simulink model "AllMethods"  (R2024a)
settings: Solver=ode4  StartTime=0.0  StopTime=40  FixedStep=dt  RelTol=1e-3
undefined symbols (not defined in the file): a0, a1, a2, a3, a4, a5, a6, a7, A_cplant, Ag, AgN, alpha1, alpha2, B_cplant, C_cplant, C_phys_5dof, CNrt, CRrt, D_cplant, Dd_ss, delay, Ds_ss, dt, dv1, dv2, EQ_intensity, EQ_sw, F, FN, Gnd_ss, Gns_ss, Hs1, Hs2, k3, k4, k6, K_lqr, K_phys_5dof, Kbar_inv, KE, KNbar_inv, Koo, Kot, l, lN, M_phys_5dof, MNrt, Mren, MRrt, Muu, Phi_u2, Rbar, RNbar, Seed_snr
libraries: simulink x4, slpidlib x4, sldrtlib x1
(part 2 of 2)

== system AllMethods/PID控制+坐标变换/坐标转换 此处将横向位移与节点转角转为 两个作动器的位移 ==
  "[x, theta]" : Inport
  Constant : Constant  Value=dv2
  Constant1 : Constant  Value=dv1
  Constant2 : Constant  Value=alpha2
  Constant3 : Constant  Value=alpha1
  Demux1 : Demux  Outputs=2
  Mux : Mux  Inputs=2
  Product : Product
  Product1 : Product
  Sum{,1,3,5} (4 alike) : Sum  Inputs=|++
  Sum2 : Sum  Inputs=|+-
  Sum4 : Sum  Inputs=|+-
  Trigonometric Function{,1..3} (4 alike) : Trigonometry  Operator=cos
  m to mm : Gain  Gain=1000
  "m to mm " : Gain  Gain=1000
  "[xa1,xa2] mm" : Outport  VectorParamsAs1DForOutWhenUnconnected=off
  wires:
  Constant/1 -> Product/1
  Constant2/1 -> Sum1/2, Trigonometric Function1/1
  Sum1/1 -> Trigonometric Function/1
  Trigonometric Function/1 -> Sum2/1
  Trigonometric Function1/1 -> Sum2/2
  Sum2/1 -> Product/2
  Product/1 -> Sum/2
  Sum/1 -> m to mm/1
  Sum4/1 -> Product1/2
  Trigonometric Function3/1 -> Sum4/2
  Trigonometric Function2/1 -> Sum4/1
  Sum3/1 -> Trigonometric Function2/1
  Constant3/1 -> Sum3/2, Trigonometric Function3/1
  Constant1/1 -> Product1/1
  Product1/1 -> Sum5/2
  Sum5/1 -> "m to mm "/1
  "m to mm "/1 -> Mux/1  "xa1 (mm)"
  m to mm/1 -> Mux/2  "xa2 (mm)"
  Demux1/1 -> Sum/1, Sum5/1  "x (m)"
  "[x, theta]"/1 -> Demux1/1
  Demux1/2 -> Sum3/1, Sum1/1  "theta (rad)"
  Mux/1 -> "[xa1,xa2] mm"/1

== system AllMethods/PID控制+坐标变换/控制器与作动器 ==
  Target actuator displacement vector (mm) : Inport
  Control Plant4 : StateSpace  A=A_cplant  B=B_cplant  C=C_cplant  D=D_cplant  InitialCondition=0
  Delay : Delay  DelayLength=37
  Demux7 : Demux  Outputs=2
  Mux4 : Mux  Inputs=2
  PID Controller2 : slpidlib/PID Controller  Controller=PID  Form=Parallel  TimeDomain=Discrete-time  UseExternalTs=off  SampleTime=-1  IntegratorMethod=Forward Euler  FilterMethod=Forward Euler  ControllerParametersSource=internal  P=1  I=50  UseKiTs=off  D=1e-10  UseExternalDerivativeSource=off  N=100  UseFilter=off  TunerSelectOption=Transfer Function Based (PID Tuner App)  InitialConditionSource=internal  InitialConditionForIntegrator=0  InitialConditionForFilter=0  DifferentiatorICPrevScaledInput=0  ExternalReset=none  TrackingMode=off  Kt=1  LimitOutput=off  SatLimitsSource=internal  UpperSaturationLimit=inf  LowerSaturationLimit=-inf  LinearizeAsGain=on  AntiWindupMode=none  Kb=1  LimitIntegrator=off  UpperIntegratorSaturationLimit=inf  LowerIntegratorSaturationLimit=-inf  POutMin=[]  POutMax=[]  IOutMin=[]  IOutMax=[]  DOutMin=[]  DOutMax=[]  NOutMin=[]  NOutMax=[]  SumOutMin=[]  SumOutMax=[]  SaturationOutMin=[]  SaturationOutMax=[]  PParamMin=[]  PParamMax=[]  IParamMin=[]  IParamMax=[]  DParamMin=[]  DParamMax=[]  NParamMin=[]  NParamMax=[]  KbParamMin=[]  KbParamMax=[]  KtParamMin=[]  KtParamMax=[]  KbOutMin=[]  KbOutMax=[]  KtOutMin=[]  KtOutMax=[]  IntegratorOutMin=[]  IntegratorOutMax=[]  FilterOutMin=[]  FilterOutMax=[]  SumI1OutMin=[]  SumI1OutMax=[]  SumI2OutMin=[]  SumI2OutMax=[]  SumI3OutMin=[]  SumI3OutMax=[]  SumI4OutMin=[]  SumI4OutMax=[]  SumDOutMin=[]  SumDOutMax=[]  DifferentiatorOutMin=[]  DifferentiatorOutMax=[]  FilterDiffOutCoefMin=[]  FilterDiffOutCoefMax=[]  ReciprocalOutMin=[]  ReciprocalOutMax=[]  SumDenOutMin=[]  SumDenOutMax=[]  SumNumOutMin=[]  SumNumOutMax=[]  DivideOutMin=[]  DivideOutMax=[]  UdiffTsProdOutMin=[]  UdiffTsProdOutMax=[]  NTsProdOutMin=[]  NTsProdOutMax=[]  UintegralTsProdOutMin=[]  UintegralTsProdOutMax=[]  UngainTsProdOutMin=[]  UngainTsProdOutMax=[]  ClampingZeroOutDataTypeStr=Inherit: Inherit via back propagation  ClampingZeroOutMin=[]  ClampingZeroOutMax=[]  FilterDenConstantOutDataTypeStr=Inherit: Inherit via back propagation  FilterDenConstantOutMin=[]  FilterDenConstantOutMax=[]  PCopyOutDataTypeStr=Inherit: Inherit via back propagation  PCopyOutMin=[]  PCopyOutMax=[]  NCopyOutDataTypeStr=Inherit: Inherit via back propagation  NCopyOutMin=[]  NCopyOutMax=[]  IntegratorContinuousStateAttributes=''  IntegratorStateMustResolveToSignalObject=off  IntegratorRTWStateStorageClass=Auto  FilterContinuousStateAttributes=''  FilterStateMustResolveToSignalObject=off  FilterRTWStateStorageClass=Auto  ParallelPVariant=InternalParameters  IdealPVariant=Disabled  IVariant=InternalParameters  DVariant=InternalParameters  IntegratorVariant=Discrete  SatVariant=Disabled  AWVariant=Passthrough  PCopyVariant=Disabled  TRVariant=Disabled  FdbkBlocksVariant=Forward  IdealPFdbkVariant=Disabled  SatFdbkVariant=Disabled  DerivativeFilterVariant=Differentiator  NVariant=Passthrough  NCopyVariant=Disabled_SignalSpec  FilterICVariant=InternalICsDifferentiator  IntegratorICVariant=InternalICs  ExternalResetVariant=Disabled  TRSumVariant=Passthrough  SumFdbkVariant=Disabled  SumVariant=Sum_PID  TsampFilterVariant=InternalTs  TsampNgainVariant=Passthrough  TsampIntegralVariant=Disabled_SignalSpec  ExternalSaturationOutDataTypeStr=Inherit: Same as second input  DerivativeSourceVariant=ErrorSignal
  PID Controller4 : slpidlib/PID Controller  Controller=PID  Form=Parallel  TimeDomain=Discrete-time  UseExternalTs=off  SampleTime=-1  IntegratorMethod=Forward Euler  FilterMethod=Forward Euler  ControllerParametersSource=internal  P=1  I=50  UseKiTs=off  D=1e-10  UseExternalDerivativeSource=off  N=100  UseFilter=on  TunerSelectOption=Transfer Function Based (PID Tuner App)  InitialConditionSource=internal  InitialConditionForIntegrator=0  InitialConditionForFilter=0  DifferentiatorICPrevScaledInput=0  ExternalReset=none  TrackingMode=off  Kt=1  LimitOutput=off  SatLimitsSource=internal  UpperSaturationLimit=inf  LowerSaturationLimit=-inf  LinearizeAsGain=on  AntiWindupMode=none  Kb=1  LimitIntegrator=off  UpperIntegratorSaturationLimit=inf  LowerIntegratorSaturationLimit=-inf  POutMin=[]  POutMax=[]  IOutMin=[]  IOutMax=[]  DOutMin=[]  DOutMax=[]  NOutMin=[]  NOutMax=[]  SumOutMin=[]  SumOutMax=[]  SaturationOutMin=[]  SaturationOutMax=[]  PParamMin=[]  PParamMax=[]  IParamMin=[]  IParamMax=[]  DParamMin=[]  DParamMax=[]  NParamMin=[]  NParamMax=[]  KbParamMin=[]  KbParamMax=[]  KtParamMin=[]  KtParamMax=[]  KbOutMin=[]  KbOutMax=[]  KtOutMin=[]  KtOutMax=[]  IntegratorOutMin=[]  IntegratorOutMax=[]  FilterOutMin=[]  FilterOutMax=[]  SumI1OutMin=[]  SumI1OutMax=[]  SumI2OutMin=[]  SumI2OutMax=[]  SumI3OutMin=[]  SumI3OutMax=[]  SumI4OutMin=[]  SumI4OutMax=[]  SumDOutMin=[]  SumDOutMax=[]  DifferentiatorOutMin=[]  DifferentiatorOutMax=[]  FilterDiffOutCoefMin=[]  FilterDiffOutCoefMax=[]  ReciprocalOutMin=[]  ReciprocalOutMax=[]  SumDenOutMin=[]  SumDenOutMax=[]  SumNumOutMin=[]  SumNumOutMax=[]  DivideOutMin=[]  DivideOutMax=[]  UdiffTsProdOutMin=[]  UdiffTsProdOutMax=[]  NTsProdOutMin=[]  NTsProdOutMax=[]  UintegralTsProdOutMin=[]  UintegralTsProdOutMax=[]  UngainTsProdOutMin=[]  UngainTsProdOutMax=[]  ClampingZeroOutDataTypeStr=Inherit: Inherit via back propagation  ClampingZeroOutMin=[]  ClampingZeroOutMax=[]  FilterDenConstantOutDataTypeStr=Inherit: Inherit via back propagation  FilterDenConstantOutMin=[]  FilterDenConstantOutMax=[]  PCopyOutDataTypeStr=Inherit: Inherit via back propagation  PCopyOutMin=[]  PCopyOutMax=[]  NCopyOutDataTypeStr=Inherit: Inherit via back propagation  NCopyOutMin=[]  NCopyOutMax=[]  IntegratorContinuousStateAttributes=''  IntegratorStateMustResolveToSignalObject=off  IntegratorRTWStateStorageClass=Auto  FilterContinuousStateAttributes=''  FilterStateMustResolveToSignalObject=off  FilterRTWStateStorageClass=Auto  ParallelPVariant=InternalParameters  IdealPVariant=Disabled  IVariant=InternalParameters  DVariant=InternalParameters  IntegratorVariant=Discrete  SatVariant=Disabled  AWVariant=Passthrough  PCopyVariant=Disabled  TRVariant=Disabled  FdbkBlocksVariant=Forward  IdealPFdbkVariant=Disabled  SatFdbkVariant=Disabled  DerivativeFilterVariant=ForwardEulerFilter  NVariant=InternalParameters  NCopyVariant=Disabled  FilterICVariant=InternalICsFilter  IntegratorICVariant=InternalICs  ExternalResetVariant=Disabled  TRSumVariant=Passthrough  SumFdbkVariant=Disabled  SumVariant=Sum_PID  TsampFilterVariant=InternalTs  TsampNgainVariant=Passthrough  TsampIntegralVariant=Disabled_SignalSpec  ExternalSaturationOutDataTypeStr=Inherit: Same as second input  DerivativeSourceVariant=ErrorSignal
  Sum11 : Sum  Inputs=|+-
  Filtered actuator displacement vector : Outport
  wires:
  PID Controller4/1 -> Mux4/2
  Control Plant4/1 -> Delay/1, Filtered actuator displacement vector/1  "Filtered actuator displacement vector"
  Sum11/1 -> Demux7/1
  PID Controller2/1 -> Mux4/1
  Mux4/1 -> Control Plant4/1
  Target actuator displacement vector (mm)/1 -> Sum11/1
  Demux7/1 -> PID Controller2/1
  Demux7/2 -> PID Controller4/1
  Delay/1 -> Sum11/2

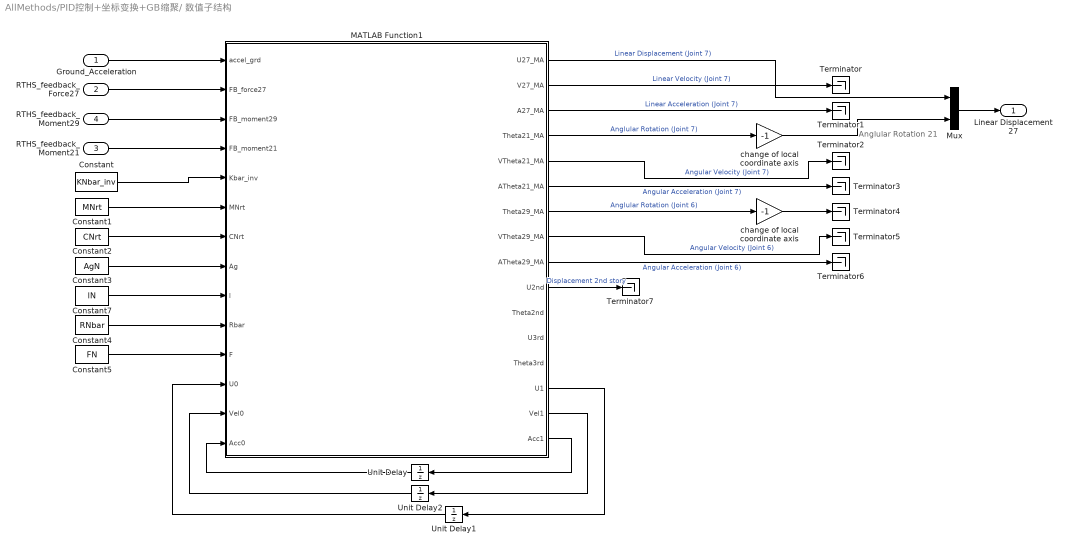
== system AllMethods/PID控制+坐标变换+GB缩聚/ 数值子结构 ==
  note: Anglular Rotation 21
  Ground_Acceleration : Inport
  RTHS_feedback_Force27 : Inport  Port=2
  RTHS_feedback_Moment21 : Inport  Port=3
  RTHS_feedback_Moment29 : Inport  Port=4
  Constant : Constant  Value=KNbar_inv  VectorParams1D=off
  Constant1 : Constant  Value=MNrt  VectorParams1D=off
  Constant2 : Constant  Value=CNrt  VectorParams1D=off
  Constant3 : Constant  Value=AgN  VectorParams1D=off
  Constant4 : Constant  Value=RNbar  VectorParams1D=off
  Constant5 : Constant  Value=FN  VectorParams1D=off
  Constant7 : Constant  Value=lN  VectorParams1D=off
  MATLAB Function1 : MATLAB Function  TreatAsAtomicUnit=on
  Mux : Mux  Inputs=2
  Terminator{,1..7} (8 alike) : Terminator
  Unit Delay : UnitDelay  SampleTime=-1  HasFrameUpgradeWarning=on
  Unit Delay1 : UnitDelay  SampleTime=-1  HasFrameUpgradeWarning=on
  Unit Delay2 : UnitDelay  SampleTime=-1  HasFrameUpgradeWarning=on
  change of local coordinate axis : Gain  Gain=-1
  "change of local coordinate axis  " : Gain  Gain=-1
  Linear Displacement 27 : Outport  VectorParamsAs1DForOutWhenUnconnected=off
  wires:
  Ground_Acceleration/1 -> MATLAB Function1/1(accel_grd)
  RTHS_feedback_Force27/1 -> MATLAB Function1/2(FB_force27)
  RTHS_feedback_Moment29/1 -> MATLAB Function1/3(FB_moment29)
  MATLAB Function1/1(U27_MA) -> Mux/1  "Linear Displacement (Joint 7)"
  MATLAB Function1/4(Theta21_MA) -> change of local coordinate axis/1  "Anglular Rotation (Joint 7)"
  Constant/1 -> MATLAB Function1/5(Kbar_inv)
  Constant1/1 -> MATLAB Function1/6(MNrt)
  Constant2/1 -> MATLAB Function1/7(CNrt)
  Constant3/1 -> MATLAB Function1/8(Ag)
  Constant7/1 -> MATLAB Function1/9(l)
  Constant4/1 -> MATLAB Function1/10(Rbar)
  Unit Delay1/1 -> MATLAB Function1/12(U0)
  Unit Delay2/1 -> MATLAB Function1/13(Vel0)
  Unit Delay/1 -> MATLAB Function1/14(Acc0)
  MATLAB Function1/15(Vel1) -> Unit Delay2/1
  MATLAB Function1/16(Acc1) -> Unit Delay/1
  MATLAB Function1/14(U1) -> Unit Delay1/1
  Constant5/1 -> MATLAB Function1/11(F)
  MATLAB Function1/2(V27_MA) -> Terminator/1  "Linear Velocity (Joint 7)"
  MATLAB Function1/3(A27_MA) -> Terminator1/1  "Linear Acceleration (Joint 7)"
  MATLAB Function1/5(VTheta21_MA) -> Terminator2/1  "Angular Velocity (Joint 7)"
  MATLAB Function1/6(ATheta21_MA) -> Terminator3/1  "Angular Acceleration (Joint 7)"
  MATLAB Function1/9(ATheta29_MA) -> Terminator6/1  "Angular Acceleration (Joint 6)"
  MATLAB Function1/8(VTheta29_MA) -> Terminator5/1  "Angular Velocity (Joint 6)"
  MATLAB Function1/7(Theta29_MA) -> "change of local coordinate axis  "/1  "Anglular Rotation (Joint 6)"
  RTHS_feedback_Moment21/1 -> MATLAB Function1/4(FB_moment21)
  change of local coordinate axis/1 -> Mux/2
  "change of local coordinate axis  "/1 -> Terminator4/1
  Mux/1 -> Linear Displacement 27/1
  MATLAB Function1/10(U2nd) -> Terminator7/1  "Displacement 2nd story"

== system AllMethods/PID控制+坐标变换+GB缩聚/Feedback Force Computation ==
  note: F(27)
  note: M(21)
  note: M(29)
  "[x_est, theta_est] (m,rad)" : Inport
  Demux : Demux  Outputs=3
  Derivative : Derivative
  Derivative1 : Derivative
  Gain1 : Gain  Gain=K_phys_5dof  Multiplication=Matrix(K*u) (u vector)
  Gain2 : Gain  Gain=C_phys_5dof  Multiplication=Matrix(K*u) (u vector)
  Gain3 : Gain  Gain=M_phys_5dof  Multiplication=Matrix(K*u) (u vector)
  Gain4 : Gain  Commented=on  Gain=-inv(Koo)*Kot  Multiplication=Matrix(K*u) (u vector)
  Mux2 : Mux  Commented=on  Inputs=2
  Mux3 : Mux  Inputs=2
  Selector : Selector  InputPortWidth=5  IndexOptions=Index vector (dialog)  Indices=[1 2 3]  OutputSizes=1
  Sum : Sum  Inputs=+|+|+
  Sum1 : Sum  Inputs=|++
  change of local coordinate axis2 : Gain  Gain=-1
  change of local coordinate axis3 : Gain  Gain=-1
  动态位移 : Gain  Gain=Phi_u2*Phi_u2' * Muu  Multiplication=Matrix(K*u) (u vector)
  静态位移 : Gain  Gain=-Kuu \ Kuc  Multiplication=Matrix(K*u) (u vector)
  F(27)_phys (N) : Outport  VectorParamsAs1DForOutWhenUnconnected=off
  M(21)_phys (N*m) : Outport  Port=2  VectorParamsAs1DForOutWhenUnconnected=off
  M(29)_phys (N*m) : Outport  Port=3  VectorParamsAs1DForOutWhenUnconnected=off
  wires:
  Derivative1/1 -> Gain3/1
  Gain2/1 -> Sum/2
  Derivative/1 -> Gain2/1, Derivative1/1
  Gain1/1 -> Sum/1
  Demux/1 -> F(27)_phys (N)/1
  Sum/1 -> Selector/1
  Selector/1 -> Demux/1
  Gain3/1 -> Sum/3
  Demux/2 -> change of local coordinate axis2/1
  Demux/3 -> change of local coordinate axis3/1
  Mux3/1 -> Derivative/1, Gain1/1
  change of local coordinate axis2/1 -> M(21)_phys (N*m)/1
  change of local coordinate axis3/1 -> M(29)_phys (N*m)/1
  静态位移/1 -> 动态位移/1, Sum1/2
  "[x_est, theta_est] (m,rad)"/1 -> Mux2/1, Gain4/1, Mux3/1, 静态位移/1
  动态位移/1 -> Sum1/1
  Gain4/1 -> Mux2/2
  Sum1/1 -> Mux3/2

== system AllMethods/PID控制+坐标变换+GB缩聚/坐标转换 此处将两个作动器的位移转为 横向位移与节点转角  ==
  "[xm1_est, xm2_est] (mm)" : Inport
  Constant : Constant  Value=dv2
  Constant1 : Constant  Value=dv1
  Constant2 : Constant  Value=alpha2
  Constant3 : Constant  Value=alpha1
  Demux1 : Demux  Outputs=2
  Divide : Product  Inputs=*/
  Gain : Gain  Gain=2
  Mux2 : Mux  Inputs=2
  Product : Product
  Product1 : Product
  Sum : Sum  Inputs=+-|
  Sum1 : Sum  Inputs=|++
  Sum2 : Sum  Inputs=|+-
  Sum3 : Sum  Inputs=-+|
  Trigonometric Function1 : Trigonometry
  Trigonometric Function2 : Trigonometry  Operator=cos
  Trigonometric Function3 : Trigonometry  Operator=cos
  Trigonometric Function4 : Trigonometry  Operator=asin
  mm to m : Gain  Gain=1/1000
  "mm to m " : Gain  Gain=1/1000
  "[x, theta] (m, rad)" : Outport  VectorParamsAs1DForOutWhenUnconnected=off
  wires:
  Constant2/1 -> Trigonometric Function1/1
  Constant1/1 -> Product1/1
  Demux1/1 -> mm to m/1
  Demux1/2 -> "mm to m "/1
  Sum/1 -> Divide/1
  Constant/1 -> Gain/1
  Trigonometric Function1/1 -> Product/2
  Gain/1 -> Product/1
  Product/1 -> Divide/2
  Divide/1 -> Sum1/2, Trigonometric Function4/1
  Sum1/1 -> Trigonometric Function2/1
  Constant3/1 -> Sum1/1, Trigonometric Function3/1
  Sum3/1 -> Product1/2
  Sum2/1 -> Mux2/1
  Trigonometric Function2/1 -> Sum3/2
  Trigonometric Function3/1 -> Sum3/1
  Product1/1 -> Sum2/2
  mm to m/1 -> Sum2/1, Sum/1
  "mm to m "/1 -> Sum/2
  Trigonometric Function4/1 -> Mux2/2
  "[xm1_est, xm2_est] (mm)"/1 -> Demux1/1
  Mux2/1 -> "[x, theta] (m, rad)"/1

== system AllMethods/PID控制+坐标变换+GB缩聚/坐标转换 此处将横向位移与节点转角转为 两个作动器的位移 ==
  "[x, theta]" : Inport
  Constant : Constant  Value=dv2
  Constant1 : Constant  Value=dv1
  Constant2 : Constant  Value=alpha2
  Constant3 : Constant  Value=alpha1
  Demux1 : Demux  Outputs=2
  Mux : Mux  Inputs=2
  Product : Product
  Product1 : Product
  Sum{,1,3,5} (4 alike) : Sum  Inputs=|++
  Sum2 : Sum  Inputs=|+-
  Sum4 : Sum  Inputs=|+-
  Trigonometric Function{,1..3} (4 alike) : Trigonometry  Operator=cos
  m to mm : Gain  Gain=1000
  "m to mm " : Gain  Gain=1000
  "[xa1,xa2] mm" : Outport  VectorParamsAs1DForOutWhenUnconnected=off
  wires:
  Constant/1 -> Product/1
  Constant2/1 -> Sum1/2, Trigonometric Function1/1
  Sum1/1 -> Trigonometric Function/1
  Trigonometric Function/1 -> Sum2/1
  Trigonometric Function1/1 -> Sum2/2
  Sum2/1 -> Product/2
  Product/1 -> Sum/2
  Sum/1 -> m to mm/1
  Sum4/1 -> Product1/2
  Trigonometric Function3/1 -> Sum4/2
  Trigonometric Function2/1 -> Sum4/1
  Sum3/1 -> Trigonometric Function2/1
  Constant3/1 -> Sum3/2, Trigonometric Function3/1
  Constant1/1 -> Product1/1
  Product1/1 -> Sum5/2
  Sum5/1 -> "m to mm "/1
  "m to mm "/1 -> Mux/1  "xa1 (mm)"
  m to mm/1 -> Mux/2  "xa2 (mm)"
  Demux1/1 -> Sum/1, Sum5/1  "x (m)"
  "[x, theta]"/1 -> Demux1/1
  Demux1/2 -> Sum3/1, Sum1/1  "theta (rad)"
  Mux/1 -> "[xa1,xa2] mm"/1

== system AllMethods/PID控制+坐标变换+GB缩聚/控制器与作动器 ==
  Target actuator displacement vector (mm) : Inport
  Control Plant4 : StateSpace  A=A_cplant  B=B_cplant  C=C_cplant  D=D_cplant  InitialCondition=0
  Delay : Delay  DelayLength=37
  Demux7 : Demux  Outputs=2
  Mux4 : Mux  Inputs=2
  PID Controller2 : slpidlib/PID Controller  Controller=PID  Form=Parallel  TimeDomain=Discrete-time  UseExternalTs=off  SampleTime=-1  IntegratorMethod=Forward Euler  FilterMethod=Forward Euler  ControllerParametersSource=internal  P=1  I=50  UseKiTs=off  D=1e-10  UseExternalDerivativeSource=off  N=100  UseFilter=off  TunerSelectOption=Transfer Function Based (PID Tuner App)  InitialConditionSource=internal  InitialConditionForIntegrator=0  InitialConditionForFilter=0  DifferentiatorICPrevScaledInput=0  ExternalReset=none  TrackingMode=off  Kt=1  LimitOutput=off  SatLimitsSource=internal  UpperSaturationLimit=inf  LowerSaturationLimit=-inf  LinearizeAsGain=on  AntiWindupMode=none  Kb=1  LimitIntegrator=off  UpperIntegratorSaturationLimit=inf  LowerIntegratorSaturationLimit=-inf  POutMin=[]  POutMax=[]  IOutMin=[]  IOutMax=[]  DOutMin=[]  DOutMax=[]  NOutMin=[]  NOutMax=[]  SumOutMin=[]  SumOutMax=[]  SaturationOutMin=[]  SaturationOutMax=[]  PParamMin=[]  PParamMax=[]  IParamMin=[]  IParamMax=[]  DParamMin=[]  DParamMax=[]  NParamMin=[]  NParamMax=[]  KbParamMin=[]  KbParamMax=[]  KtParamMin=[]  KtParamMax=[]  KbOutMin=[]  KbOutMax=[]  KtOutMin=[]  KtOutMax=[]  IntegratorOutMin=[]  IntegratorOutMax=[]  FilterOutMin=[]  FilterOutMax=[]  SumI1OutMin=[]  SumI1OutMax=[]  SumI2OutMin=[]  SumI2OutMax=[]  SumI3OutMin=[]  SumI3OutMax=[]  SumI4OutMin=[]  SumI4OutMax=[]  SumDOutMin=[]  SumDOutMax=[]  DifferentiatorOutMin=[]  DifferentiatorOutMax=[]  FilterDiffOutCoefMin=[]  FilterDiffOutCoefMax=[]  ReciprocalOutMin=[]  ReciprocalOutMax=[]  SumDenOutMin=[]  SumDenOutMax=[]  SumNumOutMin=[]  SumNumOutMax=[]  DivideOutMin=[]  DivideOutMax=[]  UdiffTsProdOutMin=[]  UdiffTsProdOutMax=[]  NTsProdOutMin=[]  NTsProdOutMax=[]  UintegralTsProdOutMin=[]  UintegralTsProdOutMax=[]  UngainTsProdOutMin=[]  UngainTsProdOutMax=[]  ClampingZeroOutDataTypeStr=Inherit: Inherit via back propagation  ClampingZeroOutMin=[]  ClampingZeroOutMax=[]  FilterDenConstantOutDataTypeStr=Inherit: Inherit via back propagation  FilterDenConstantOutMin=[]  FilterDenConstantOutMax=[]  PCopyOutDataTypeStr=Inherit: Inherit via back propagation  PCopyOutMin=[]  PCopyOutMax=[]  NCopyOutDataTypeStr=Inherit: Inherit via back propagation  NCopyOutMin=[]  NCopyOutMax=[]  IntegratorContinuousStateAttributes=''  IntegratorStateMustResolveToSignalObject=off  IntegratorRTWStateStorageClass=Auto  FilterContinuousStateAttributes=''  FilterStateMustResolveToSignalObject=off  FilterRTWStateStorageClass=Auto  ParallelPVariant=InternalParameters  IdealPVariant=Disabled  IVariant=InternalParameters  DVariant=InternalParameters  IntegratorVariant=Discrete  SatVariant=Disabled  AWVariant=Passthrough  PCopyVariant=Disabled  TRVariant=Disabled  FdbkBlocksVariant=Forward  IdealPFdbkVariant=Disabled  SatFdbkVariant=Disabled  DerivativeFilterVariant=Differentiator  NVariant=Passthrough  NCopyVariant=Disabled_SignalSpec  FilterICVariant=InternalICsDifferentiator  IntegratorICVariant=InternalICs  ExternalResetVariant=Disabled  TRSumVariant=Passthrough  SumFdbkVariant=Disabled  SumVariant=Sum_PID  TsampFilterVariant=InternalTs  TsampNgainVariant=Passthrough  TsampIntegralVariant=Disabled_SignalSpec  ExternalSaturationOutDataTypeStr=Inherit: Same as second input  DerivativeSourceVariant=ErrorSignal
  PID Controller4 : slpidlib/PID Controller  Controller=PID  Form=Parallel  TimeDomain=Discrete-time  UseExternalTs=off  SampleTime=-1  IntegratorMethod=Forward Euler  FilterMethod=Forward Euler  ControllerParametersSource=internal  P=1  I=50  UseKiTs=off  D=1e-10  UseExternalDerivativeSource=off  N=100  UseFilter=on  TunerSelectOption=Transfer Function Based (PID Tuner App)  InitialConditionSource=internal  InitialConditionForIntegrator=0  InitialConditionForFilter=0  DifferentiatorICPrevScaledInput=0  ExternalReset=none  TrackingMode=off  Kt=1  LimitOutput=off  SatLimitsSource=internal  UpperSaturationLimit=inf  LowerSaturationLimit=-inf  LinearizeAsGain=on  AntiWindupMode=none  Kb=1  LimitIntegrator=off  UpperIntegratorSaturationLimit=inf  LowerIntegratorSaturationLimit=-inf  POutMin=[]  POutMax=[]  IOutMin=[]  IOutMax=[]  DOutMin=[]  DOutMax=[]  NOutMin=[]  NOutMax=[]  SumOutMin=[]  SumOutMax=[]  SaturationOutMin=[]  SaturationOutMax=[]  PParamMin=[]  PParamMax=[]  IParamMin=[]  IParamMax=[]  DParamMin=[]  DParamMax=[]  NParamMin=[]  NParamMax=[]  KbParamMin=[]  KbParamMax=[]  KtParamMin=[]  KtParamMax=[]  KbOutMin=[]  KbOutMax=[]  KtOutMin=[]  KtOutMax=[]  IntegratorOutMin=[]  IntegratorOutMax=[]  FilterOutMin=[]  FilterOutMax=[]  SumI1OutMin=[]  SumI1OutMax=[]  SumI2OutMin=[]  SumI2OutMax=[]  SumI3OutMin=[]  SumI3OutMax=[]  SumI4OutMin=[]  SumI4OutMax=[]  SumDOutMin=[]  SumDOutMax=[]  DifferentiatorOutMin=[]  DifferentiatorOutMax=[]  FilterDiffOutCoefMin=[]  FilterDiffOutCoefMax=[]  ReciprocalOutMin=[]  ReciprocalOutMax=[]  SumDenOutMin=[]  SumDenOutMax=[]  SumNumOutMin=[]  SumNumOutMax=[]  DivideOutMin=[]  DivideOutMax=[]  UdiffTsProdOutMin=[]  UdiffTsProdOutMax=[]  NTsProdOutMin=[]  NTsProdOutMax=[]  UintegralTsProdOutMin=[]  UintegralTsProdOutMax=[]  UngainTsProdOutMin=[]  UngainTsProdOutMax=[]  ClampingZeroOutDataTypeStr=Inherit: Inherit via back propagation  ClampingZeroOutMin=[]  ClampingZeroOutMax=[]  FilterDenConstantOutDataTypeStr=Inherit: Inherit via back propagation  FilterDenConstantOutMin=[]  FilterDenConstantOutMax=[]  PCopyOutDataTypeStr=Inherit: Inherit via back propagation  PCopyOutMin=[]  PCopyOutMax=[]  NCopyOutDataTypeStr=Inherit: Inherit via back propagation  NCopyOutMin=[]  NCopyOutMax=[]  IntegratorContinuousStateAttributes=''  IntegratorStateMustResolveToSignalObject=off  IntegratorRTWStateStorageClass=Auto  FilterContinuousStateAttributes=''  FilterStateMustResolveToSignalObject=off  FilterRTWStateStorageClass=Auto  ParallelPVariant=InternalParameters  IdealPVariant=Disabled  IVariant=InternalParameters  DVariant=InternalParameters  IntegratorVariant=Discrete  SatVariant=Disabled  AWVariant=Passthrough  PCopyVariant=Disabled  TRVariant=Disabled  FdbkBlocksVariant=Forward  IdealPFdbkVariant=Disabled  SatFdbkVariant=Disabled  DerivativeFilterVariant=ForwardEulerFilter  NVariant=InternalParameters  NCopyVariant=Disabled  FilterICVariant=InternalICsFilter  IntegratorICVariant=InternalICs  ExternalResetVariant=Disabled  TRSumVariant=Passthrough  SumFdbkVariant=Disabled  SumVariant=Sum_PID  TsampFilterVariant=InternalTs  TsampNgainVariant=Passthrough  TsampIntegralVariant=Disabled_SignalSpec  ExternalSaturationOutDataTypeStr=Inherit: Same as second input  DerivativeSourceVariant=ErrorSignal
  Sum11 : Sum  Inputs=|+-
  Filtered actuator displacement vector : Outport
  wires:
  PID Controller4/1 -> Mux4/2
  Control Plant4/1 -> Delay/1, Filtered actuator displacement vector/1  "Filtered actuator displacement vector"
  Sum11/1 -> Demux7/1
  PID Controller2/1 -> Mux4/1
  Mux4/1 -> Control Plant4/1
  Target actuator displacement vector (mm)/1 -> Sum11/1
  Demux7/1 -> PID Controller2/1
  Demux7/2 -> PID Controller4/1
  Delay/1 -> Sum11/2

== system AllMethods/离散时间下封装模块/Feedback Force Computation ==
  "[x_est, theta_est] (m,rad)" : Inport
  Derivative : Derivative
  Derivative1 : Derivative
  Gain1 : Gain  Gain=K_phys_5dof  Multiplication=Matrix(K*u) (u vector)
  Gain2 : Gain  Gain=C_phys_5dof  Multiplication=Matrix(K*u) (u vector)
  Gain3 : Gain  Gain=M_phys_5dof  Multiplication=Matrix(K*u) (u vector)
  Sum : Sum  Inputs=+|+|+
  F(27)_phys (N) : Outport  VectorParamsAs1DForOutWhenUnconnected=off
  wires:
  Derivative1/1 -> Gain3/1
  Gain2/1 -> Sum/2
  Derivative/1 -> Gain2/1, Derivative1/1
  Gain1/1 -> Sum/1
  Sum/1 -> F(27)_phys (N)/1
  Gain3/1 -> Sum/3
  "[x_est, theta_est] (m,rad)"/1 -> Derivative/1, Gain1/1

== system AllMethods/连续时间下封装模块/Feedback Force Computation1 ==
  "[x_est, theta_est] (m,rad)" : Inport
  Derivative : Derivative
  Derivative1 : Derivative
  Gain1 : Gain  Gain=K_phys_5dof  Multiplication=Matrix(K*u) (u vector)
  Gain2 : Gain  Gain=C_phys_5dof  Multiplication=Matrix(K*u) (u vector)
  Gain3 : Gain  Gain=M_phys_5dof  Multiplication=Matrix(K*u) (u vector)
  Sum : Sum  Inputs=+|+|+
  F(27)_phys (N) : Outport  VectorParamsAs1DForOutWhenUnconnected=off
  wires:
  Derivative1/1 -> Gain3/1
  Gain2/1 -> Sum/2
  Derivative/1 -> Gain2/1, Derivative1/1
  Gain1/1 -> Sum/1
  Sum/1 -> F(27)_phys (N)/1
  Gain3/1 -> Sum/3
  "[x_est, theta_est] (m,rad)"/1 -> Derivative/1, Gain1/1

== matlab function AllMethods/LQG+坐标变换+GB缩聚/ NUMERICAL SUBSTRUCTURE/MATLAB Function1 ==
  data: U27_MA output; V27_MA output; A27_MA output; Theta21_MA output; VTheta21_MA output; ATheta21_MA output; Theta29_MA output; VTheta29_MA output; ATheta29_MA output; U2nd output; Theta2nd output; U3rd output; Theta3rd output; U1 output; Vel1 output; Acc1 output; accel_grd input; FB_force27 input; FB_moment29 input; FB_moment21 input; Kbar_inv input; MNrt input; CNrt input; Ag input; l input; Rbar input; F input; U0 input; Vel0 input; Acc0 input; a0 parameter; a1 parameter; a2 parameter; a3 parameter; a4 parameter; a5 parameter; a6 parameter; a7 parameter
function [U27_MA,V27_MA,A27_MA,Theta21_MA,VTheta21_MA,ATheta21_MA,Theta29_MA,VTheta29_MA,ATheta29_MA,U2nd,Theta2nd,U3rd,Theta3rd,U1,Vel1,Acc1]=...
    fcn(accel_grd,FB_force27,FB_moment29,FB_moment21,Kbar_inv, MNrt, CNrt,Ag,l,Rbar,F,...
    U0,Vel0,Acc0, a0, a1, a2, a3, a4, a5, a6, a7)
             
             
    % ============================
	% *  Update next iteration   *
	% ============================
    ndof = length(Kbar_inv);
    U1   = zeros(ndof,1);
    Vel1 = zeros(ndof,1);
    Acc1 = zeros(ndof,1);
    
    U27_MA = 0;
    V27_MA = 0;
    A27_MA = 0;

    Theta21_MA = 0;
    VTheta21_MA = 0;
    ATheta21_MA = 0;
% 
%     U6_MA = 0;
%     V6_MA = 0;
%     A6_MA = 0;
    U2nd = 0 ;              %Displacement 2nd story, node 12, DOF 26
    Theta2nd = 0;          %Rotation 2nd story, node 12, DOF 22
    U3rd = 0;              %Displacement 3rd story, node 16, DOF 13
    Theta3rd = 0;           %Rotation 3rd story, node 16, DOF 3


    Theta29_MA = 0;
    VTheta29_MA = 0;
    ATheta29_MA = 0;

    % ============================
	% *  Feedback Force / Moment *
	% ============================
    F(27) = FB_force27;
    F(21) = FB_moment21;
    F(29) = FB_moment29;

    % ==========================
	% *     Update Matrices    *
	% ==========================
    Ag(:)  = accel_grd * l;
    
   	% ==========================
	% * 	  Form Rbar  	   *
	% ==========================
	Rbar = ( (MNrt * ((a0*U0)+(a2*Vel0)+(a3*Acc0))) + ...
		     (CNrt * ((a1*U0)+(a4*Vel0)+(a5*Acc0))) - F - (MNrt * Ag) );
    
    % ==========================
	% * Solve for Displacement *
	% ==========================
	U1 = Kbar_inv * Rbar;
    
	% ============================
	% * Compute Velocity & Accel *
	% ============================
	Acc1=a0*(U1-U0)-a2*Vel0-a3*Acc0;
	Vel1=Vel0+a7*Acc1+a6*Acc0; 

	% ============================
	% *    Output u1 and theta   *
	% ============================
    U27_MA    = U1(27);
    V27_MA    = Vel1(27);
    A27_MA    = Acc1(27);    

%     U6_MA    = U1(27);
%     V6_MA    = Vel1(27);
%     A6_MA    = Acc1(27);

    Theta21_MA = U1(21);
    VTheta21_MA = Vel1(21);
    ATheta21_MA = Acc1(21);

    Theta29_MA = U1(29);
    VTheta29_MA = Vel1(29);
    ATheta29_MA = Acc1(29);
    
    % ADDED by Johnny
    U2nd = U1(26);              %Displacement 2nd story, node 12, DOF 26
    Theta2nd = U1(22);          %Rotation 2nd story, node 12, DOF 22
    U3rd = U1(13);              %Displacement 3rd story, node 16, DOF 13
    Theta3rd = U1(3);           %Rotation 3rd story, node 16, DOF 3

end

== matlab function AllMethods/LQG+坐标变换/ NUMERICAL SUBSTRUCTURE/MATLAB Function1 ==
  data: U27_MA output; V27_MA output; A27_MA output; Theta21_MA output; VTheta21_MA output; ATheta21_MA output; Theta29_MA output; VTheta29_MA output; ATheta29_MA output; U2nd output; Theta2nd output; U3rd output; Theta3rd output; U1 output; Vel1 output; Acc1 output; accel_grd input; FB_force27 input; FB_moment29 input; FB_moment21 input; Kbar_inv input; MNrt input; CNrt input; Ag input; l input; Rbar input; F input; U0 input; Vel0 input; Acc0 input; a0 parameter; a1 parameter; a2 parameter; a3 parameter; a4 parameter; a5 parameter; a6 parameter; a7 parameter
function [U27_MA,V27_MA,A27_MA,Theta21_MA,VTheta21_MA,ATheta21_MA,Theta29_MA,VTheta29_MA,ATheta29_MA,U2nd,Theta2nd,U3rd,Theta3rd,U1,Vel1,Acc1]=...
    fcn(accel_grd,FB_force27,FB_moment29,FB_moment21,Kbar_inv, MNrt, CNrt,Ag,l,Rbar,F,...
    U0,Vel0,Acc0, a0, a1, a2, a3, a4, a5, a6, a7)
             
             
    % ============================
	% *  Update next iteration   *
	% ============================
    ndof = length(Kbar_inv);
    U1   = zeros(ndof,1);
    Vel1 = zeros(ndof,1);
    Acc1 = zeros(ndof,1);
    
    U27_MA = 0;
    V27_MA = 0;
    A27_MA = 0;

    Theta21_MA = 0;
    VTheta21_MA = 0;
    ATheta21_MA = 0;
% 
%     U6_MA = 0;
%     V6_MA = 0;
%     A6_MA = 0;
    U2nd = 0 ;              %Displacement 2nd story, node 12, DOF 26
    Theta2nd = 0;          %Rotation 2nd story, node 12, DOF 22
    U3rd = 0;              %Displacement 3rd story, node 16, DOF 13
    Theta3rd = 0;           %Rotation 3rd story, node 16, DOF 3


    Theta29_MA = 0;
    VTheta29_MA = 0;
    ATheta29_MA = 0;

    % ============================
	% *  Feedback Force / Moment *
	% ============================
    F(27) = FB_force27;
    F(21) = FB_moment21;
    F(29) = FB_moment29;

    % ==========================
	% *     Update Matrices    *
	% ==========================
    Ag(:)  = accel_grd * l;
    
   	% ==========================
	% * 	  Form Rbar  	   *
	% ==========================
	Rbar = ( (MNrt * ((a0*U0)+(a2*Vel0)+(a3*Acc0))) + ...
		     (CNrt * ((a1*U0)+(a4*Vel0)+(a5*Acc0))) - F - (MNrt * Ag) );
    
    % ==========================
	% * Solve for Displacement *
	% ==========================
	U1 = Kbar_inv * Rbar;
    
	% ============================
	% * Compute Velocity & Accel *
	% ============================
	Acc1=a0*(U1-U0)-a2*Vel0-a3*Acc0;
	Vel1=Vel0+a7*Acc1+a6*Acc0; 

	% ============================
	% *    Output u1 and theta   *
	% ============================
    U27_MA    = U1(27);
    V27_MA    = Vel1(27);
    A27_MA    = Acc1(27);    

%     U6_MA    = U1(27);
%     V6_MA    = Vel1(27);
%     A6_MA    = Acc1(27);

    Theta21_MA = U1(21);
    VTheta21_MA = Vel1(21);
    ATheta21_MA = Acc1(21);

    Theta29_MA = U1(29);
    VTheta29_MA = Vel1(29);
    ATheta29_MA = Acc1(29);
    
    % ADDED by Johnny
    U2nd = U1(26);              %Displacement 2nd story, node 12, DOF 26
    Theta2nd = U1(22);          %Rotation 2nd story, node 12, DOF 22
    U3rd = U1(13);              %Displacement 3rd story, node 16, DOF 13
    Theta3rd = U1(3);           %Rotation 3rd story, node 16, DOF 3

end

== matlab function AllMethods/PID控制+坐标变换+GB缩聚/ 数值子结构/MATLAB Function1 ==
  data: U27_MA output; V27_MA output; A27_MA output; Theta21_MA output; VTheta21_MA output; ATheta21_MA output; Theta29_MA output; VTheta29_MA output; ATheta29_MA output; U2nd output; Theta2nd output; U3rd output; Theta3rd output; U1 output; Vel1 output; Acc1 output; accel_grd input; FB_force27 input; FB_moment29 input; FB_moment21 input; Kbar_inv input; MNrt input; CNrt input; Ag input; l input; Rbar input; F input; U0 input; Vel0 input; Acc0 input; a0 parameter; a1 parameter; a2 parameter; a3 parameter; a4 parameter; a5 parameter; a6 parameter; a7 parameter
function [U27_MA,V27_MA,A27_MA,Theta21_MA,VTheta21_MA,ATheta21_MA,Theta29_MA,VTheta29_MA,ATheta29_MA,U2nd,Theta2nd,U3rd,Theta3rd,U1,Vel1,Acc1]=...
    fcn(accel_grd,FB_force27,FB_moment29,FB_moment21,Kbar_inv, MNrt, CNrt,Ag,l,Rbar,F,...
    U0,Vel0,Acc0, a0, a1, a2, a3, a4, a5, a6, a7)
             
             
    % ============================
	% *  Update next iteration   *
	% ============================
    ndof = length(Kbar_inv);
    U1   = zeros(ndof,1);
    Vel1 = zeros(ndof,1);
    Acc1 = zeros(ndof,1);
    
    U27_MA = 0;
    V27_MA = 0;
    A27_MA = 0;

    Theta21_MA = 0;
    VTheta21_MA = 0;
    ATheta21_MA = 0;
% 
%     U6_MA = 0;
%     V6_MA = 0;
%     A6_MA = 0;
    U2nd = 0 ;              %Displacement 2nd story, node 12, DOF 26
    Theta2nd = 0;          %Rotation 2nd story, node 12, DOF 22
    U3rd = 0;              %Displacement 3rd story, node 16, DOF 13
    Theta3rd = 0;           %Rotation 3rd story, node 16, DOF 3


    Theta29_MA = 0;
    VTheta29_MA = 0;
    ATheta29_MA = 0;

    % ============================
	% *  Feedback Force / Moment *
	% ============================
    F(27) = FB_force27;
    F(21) = FB_moment21;
    F(29) = FB_moment29;

    % ==========================
	% *     Update Matrices    *
	% ==========================
    Ag(:)  = accel_grd * l;
    
   	% ==========================
	% * 	  Form Rbar  	   *
	% ==========================
	Rbar = ( (MNrt * ((a0*U0)+(a2*Vel0)+(a3*Acc0))) + ...
		     (CNrt * ((a1*U0)+(a4*Vel0)+(a5*Acc0))) - F - (MNrt * Ag) );
    
    % ==========================
	% * Solve for Displacement *
	% ==========================
	U1 = Kbar_inv * Rbar;
    
	% ============================
	% * Compute Velocity & Accel *
	% ============================
	Acc1=a0*(U1-U0)-a2*Vel0-a3*Acc0;
	Vel1=Vel0+a7*Acc1+a6*Acc0; 

	% ============================
	% *    Output u1 and theta   *
	% ============================
    U27_MA    = U1(27);
    V27_MA    = Vel1(27);
    A27_MA    = Acc1(27);    

%     U6_MA    = U1(27);
%     V6_MA    = Vel1(27);
%     A6_MA    = Acc1(27);

    Theta21_MA = U1(21);
    VTheta21_MA = Vel1(21);
    ATheta21_MA = Acc1(21);

    Theta29_MA = U1(29);
    VTheta29_MA = Vel1(29);
    ATheta29_MA = Acc1(29);
    
    % ADDED by Johnny
    U2nd = U1(26);              %Displacement 2nd story, node 12, DOF 26
    Theta2nd = U1(22);          %Rotation 2nd story, node 12, DOF 22
    U3rd = U1(13);              %Displacement 3rd story, node 16, DOF 13
    Theta3rd = U1(3);           %Rotation 3rd story, node 16, DOF 3

end

== matlab function AllMethods/ REFERENCE STRUCTURE/MATLAB Function1 ==
  data: U1_MA output; Theta_MA output; U2nd output; Theta2nd output; U3rd output; Theta3rd output; ThetaNode2 output; U1 output; Vel1 output; Acc1 output; accel_grd input; Kbar_inv input; MNrt input; CNrt input; Ag input; l input; Rbar input; F input; U0 input; Vel0 input; Acc0 input; a0 parameter; a1 parameter; a2 parameter; a3 parameter; a4 parameter; a5 parameter; a6 parameter; a7 parameter; FRef output; M1Ref output; M2Ref output
function [U1_MA,Theta_MA,U2nd,Theta2nd,U3rd,Theta3rd,ThetaNode2, U1,Vel1,Acc1,FRef,M1Ref,M2Ref]=fcn(accel_grd,Kbar_inv, MNrt, CNrt,Ag,l,Rbar,F,...
    U0,Vel0,Acc0, a0, a1, a2, a3, a4, a5, a6, a7)
             
             
    % ============================
	% *  Update next iteration   *
	% ============================
    ndof = length(Kbar_inv);
    U1   = zeros(ndof,1);
    Vel1 = zeros(ndof,1);
    Acc1 = zeros(ndof,1);
    U1_MA = 0;
    Theta_MA = 0;
    FRef = 0;
    M1Ref = 0;
    M2Ref = 0;

     U2nd= 0;
    Theta2nd= 0;
    U3rd=0;
    Theta3rd=0;
    ThetaNode2=0;
    
    % ============================
	% *  Feedback Force / Moment *
	% ============================
%     F(27) = -FB_force;
%     F(14) = -FB_moment;

    % ==========================
	% *     Update Matrices    *
	% ==========================
    Ag(:)  = accel_grd * l;
    
   	% ==========================
	% * 	  Form Rbar  	   *
	% ==========================
	Rbar = ( (MNrt * ((a0*U0)+(a2*Vel0)+(a3*Acc0))) + ...
		     (CNrt * ((a1*U0)+(a4*Vel0)+(a5*Acc0))) - F - (MNrt * Ag) );
    FRef = Rbar(27);
    M1Ref= Rbar(21);
    M2Ref= Rbar(29);
    % ==========================
	% * Solve for Displacement *
	% ==========================
	U1 = Kbar_inv * Rbar;
    
	% ============================
	% * Compute Velocity & Accel *
	% ============================
	Acc1=a0*(U1-U0)-a2*Vel0-a3*Acc0;
	Vel1=Vel0+a7*Acc1+a6*Acc0; 

	% ============================
	% *    Output u1 and theta   *
	% ============================
    U1_MA    = U1(27);
    Theta_MA = U1(21);

    % ============================
	% *  Upper Stories Response  *
	% ============================
    U2nd = U1(26);              %Displacement 2nd story, node 12, DOF 26
    Theta2nd = U1(22);          %Rotation 2nd story, node 12, DOF 22
    U3rd = U1(13);              %Displacement 3rd story, node 16, DOF 13
    Theta3rd = U1(3);           %Rotation 3rd story, node 16, DOF 3
    ThetaNode2 = U1(29);        %Rotation 2nd node of the common interface, node 6, DOF 29

end

== matlab function AllMethods/PID控制+坐标变换/ 数值子结构/MATLAB Function1 ==
  data: U27_MA output; V27_MA output; A27_MA output; Theta21_MA output; VTheta21_MA output; ATheta21_MA output; Theta29_MA output; VTheta29_MA output; ATheta29_MA output; U2nd output; Theta2nd output; U3rd output; Theta3rd output; U1 output; Vel1 output; Acc1 output; accel_grd input; FB_force27 input; FB_moment29 input; FB_moment21 input; Kbar_inv input; MNrt input; CNrt input; Ag input; l input; Rbar input; F input; U0 input; Vel0 input; Acc0 input; a0 parameter; a1 parameter; a2 parameter; a3 parameter; a4 parameter; a5 parameter; a6 parameter; a7 parameter
function [U27_MA,V27_MA,A27_MA,Theta21_MA,VTheta21_MA,ATheta21_MA,Theta29_MA,VTheta29_MA,ATheta29_MA,U2nd,Theta2nd,U3rd,Theta3rd,U1,Vel1,Acc1]=...
    fcn(accel_grd,FB_force27,FB_moment29,FB_moment21,Kbar_inv, MNrt, CNrt,Ag,l,Rbar,F,...
    U0,Vel0,Acc0, a0, a1, a2, a3, a4, a5, a6, a7)
             
             
    % ============================
	% *  Update next iteration   *
	% ============================
    ndof = length(Kbar_inv);
    U1   = zeros(ndof,1);
    Vel1 = zeros(ndof,1);
    Acc1 = zeros(ndof,1);
    
    U27_MA = 0;
    V27_MA = 0;
    A27_MA = 0;

    Theta21_MA = 0;
    VTheta21_MA = 0;
    ATheta21_MA = 0;
% 
%     U6_MA = 0;
%     V6_MA = 0;
%     A6_MA = 0;
    U2nd = 0 ;              %Displacement 2nd story, node 12, DOF 26
    Theta2nd = 0;          %Rotation 2nd story, node 12, DOF 22
    U3rd = 0;              %Displacement 3rd story, node 16, DOF 13
    Theta3rd = 0;           %Rotation 3rd story, node 16, DOF 3


    Theta29_MA = 0;
    VTheta29_MA = 0;
    ATheta29_MA = 0;

    % ============================
	% *  Feedback Force / Moment *
	% ============================
    F(27) = FB_force27;
    F(21) = FB_moment21;
    F(29) = FB_moment29;

    % ==========================
	% *     Update Matrices    *
	% ==========================
    Ag(:)  = accel_grd * l;
    
   	% ==========================
	% * 	  Form Rbar  	   *
	% ==========================
	Rbar = ( (MNrt * ((a0*U0)+(a2*Vel0)+(a3*Acc0))) + ...
		     (CNrt * ((a1*U0)+(a4*Vel0)+(a5*Acc0))) - F - (MNrt * Ag) );
    
    % ==========================
	% * Solve for Displacement *
	% ==========================
	U1 = Kbar_inv * Rbar;
    
	% ============================
	% * Compute Velocity & Accel *
	% ============================
	Acc1=a0*(U1-U0)-a2*Vel0-a3*Acc0;
	Vel1=Vel0+a7*Acc1+a6*Acc0; 

	% ============================
	% *    Output u1 and theta   *
	% ============================
    U27_MA    = U1(27);
    V27_MA    = Vel1(27);
    A27_MA    = Acc1(27);    

%     U6_MA    = U1(27);
%     V6_MA    = Vel1(27);
%     A6_MA    = Acc1(27);

    Theta21_MA = U1(21);
    VTheta21_MA = Vel1(21);
    ATheta21_MA = Acc1(21);

    Theta29_MA = U1(29);
    VTheta29_MA = Vel1(29);
    ATheta29_MA = Acc1(29);
    
    % ADDED by Johnny
    U2nd = U1(26);              %Displacement 2nd story, node 12, DOF 26
    Theta2nd = U1(22);          %Rotation 2nd story, node 12, DOF 22
    U3rd = U1(13);              %Displacement 3rd story, node 16, DOF 13
    Theta3rd = U1(3);           %Rotation 3rd story, node 16, DOF 3

end

== matlab function AllMethods/1阶1/ 数值子结构2/MATLAB Function1 ==
  data: U27_MA output; V27_MA output; A27_MA output; Theta21_MA output; VTheta21_MA output; ATheta21_MA output; Theta29_MA output; VTheta29_MA output; ATheta29_MA output; U2nd output; Theta2nd output; U3rd output; Theta3rd output; U1 output; Vel1 output; Acc1 output; accel_grd input; FB_force27 input; FB_moment29 input; FB_moment21 input; Kbar_inv input; MNrt input; CNrt input; Ag input; l input; Rbar input; F input; U0 input; Vel0 input; Acc0 input; a0 parameter; a1 parameter; a2 parameter; a3 parameter; a4 parameter; a5 parameter; a6 parameter; a7 parameter; Rbar output
function [U27_MA,V27_MA,A27_MA,Theta21_MA,VTheta21_MA,ATheta21_MA,Theta29_MA,VTheta29_MA,ATheta29_MA,U2nd,Theta2nd,U3rd,Theta3rd,U1,Vel1,Acc1,Rbar]=...
    fcn(accel_grd,FB_force27,FB_moment29,FB_moment21,Kbar_inv, MNrt, CNrt,Ag,l,Rbar,F,...
    U0,Vel0,Acc0, a0, a1, a2, a3, a4, a5, a6, a7)
             
             
    % ============================
	% *  Update next iteration   *
	% ============================
    ndof = length(Kbar_inv);
    U1   = zeros(ndof,1);
    Vel1 = zeros(ndof,1);
    Acc1 = zeros(ndof,1);
    
    U27_MA = 0;
    V27_MA = 0;
    A27_MA = 0;

    Theta21_MA = 0;
    VTheta21_MA = 0;
    ATheta21_MA = 0;
% 
%     U6_MA = 0;
%     V6_MA = 0;
%     A6_MA = 0;
    U2nd = 0 ;              %Displacement 2nd story, node 12, DOF 26
    Theta2nd = 0;          %Rotation 2nd story, node 12, DOF 22
    U3rd = 0;              %Displacement 3rd story, node 16, DOF 13
    Theta3rd = 0;           %Rotation 3rd story, node 16, DOF 3


    Theta29_MA = 0;
    VTheta29_MA = 0;
    ATheta29_MA = 0;

    % ============================
	% *  Feedback Force / Moment *
	% ============================
    F(27) = FB_force27;
    F(21) = FB_moment21;
    F(29) = FB_moment29;

    % ==========================
	% *     Update Matrices    *
	% ==========================
    Ag(:)  = accel_grd * l;
    
   	% ==========================
	% * 	  Form Rbar  	   *
	% ==========================
	Rbar = ( (MNrt * ((a0*U0)+(a2*Vel0)+(a3*Acc0))) + ...
		     (CNrt * ((a1*U0)+(a4*Vel0)+(a5*Acc0))) - F - (MNrt * Ag) );
    
    % ==========================
	% * Solve for Displacement *
	% ==========================
	U1 = Kbar_inv * Rbar;
    
	% ============================
	% * Compute Velocity & Accel *
	% ============================
	Acc1=a0*(U1-U0)-a2*Vel0-a3*Acc0;
	Vel1=Vel0+a7*Acc1+a6*Acc0; 

	% ============================
	% *    Output u1 and theta   *
	% ============================
    U27_MA    = U1(27);
    V27_MA    = Vel1(27);
    A27_MA    = Acc1(27);    

%     U6_MA    = U1(27);
%     V6_MA    = Vel1(27);
%     A6_MA    = Acc1(27);

    Theta21_MA = U1(21);
    VTheta21_MA = Vel1(21);
    ATheta21_MA = Acc1(21);

    Theta29_MA = U1(29);
    VTheta29_MA = Vel1(29);
    ATheta29_MA = Acc1(29);
    
    % ADDED by Johnny
    U2nd = U1(26);              %Displacement 2nd story, node 12, DOF 26
    Theta2nd = U1(22);          %Rotation 2nd story, node 12, DOF 22
    U3rd = U1(13);              %Displacement 3rd story, node 16, DOF 13
    Theta3rd = U1(3);           %Rotation 3rd story, node 16, DOF 3

end
